simulink model "CurrentControl"  (R2021b)
settings: Solver=VariableStepAuto  StartTime=0.0  StopTime=10.0  RelTol=1e-3
undefined symbols (not defined in the file or in its folder): b, Flux
settings Model: Creator=maqui  LastModifiedBy=maqui

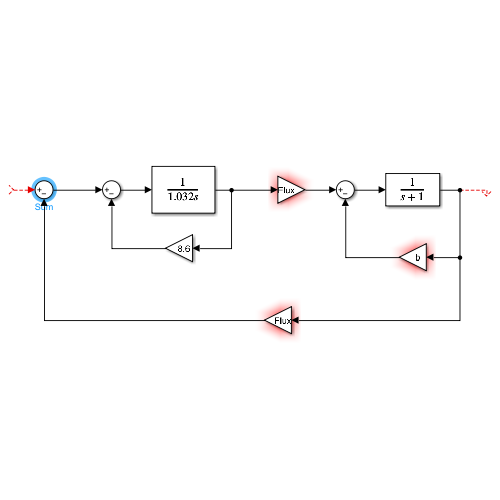
[thumbnail: Simulink's stored preview of the top-level diagram]
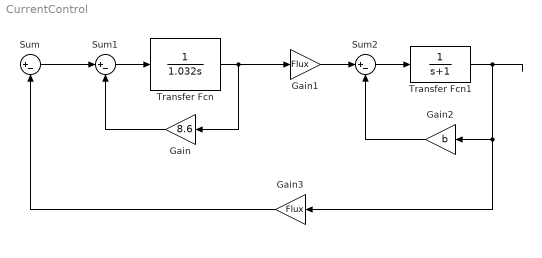
== system CurrentControl ==
  Gain : Gain  Gain=8.6
  Gain1 : Gain  Gain=Flux
  Gain2 : Gain  Gain=b
  Gain3 : Gain  Gain=Flux
  Sum : Sum  Inputs=|+-
  Sum1 : Sum  Inputs=|+-
  Sum2 : Sum  Inputs=|+-
  Transfer Fcn : TransferFcn  Denominator=[1.032 0]
  Transfer Fcn1 : TransferFcn  Denominator=[1 1]
  wires:
  Sum/1 -> Sum1/1
  Sum1/1 -> Transfer Fcn/1
  Gain/1 -> Sum1/2
  Transfer Fcn/1 -> Gain/1, Gain1/1
  Gain1/1 -> Sum2/1
  Sum2/1 -> Transfer Fcn1/1
  Transfer Fcn1/1 -> Gain3/1, Gain2/1
  Gain2/1 -> Sum2/2
  Gain3/1 -> Sum/2
  ? -> Sum/1
